simulink model "FCR_sharing"  (R2018a)
settings: Solver=VariableStepAuto  StartTime=0.0  StopTime=25  MaxStep=0.01  RelTol=1e-3
undefined symbols (not defined in the file): Fn, KESS, KGT, Sn, StepMW, Tess, Tgov1, Tgov2
settings Model: Creator=daniemot  LastModifiedBy=daniemot

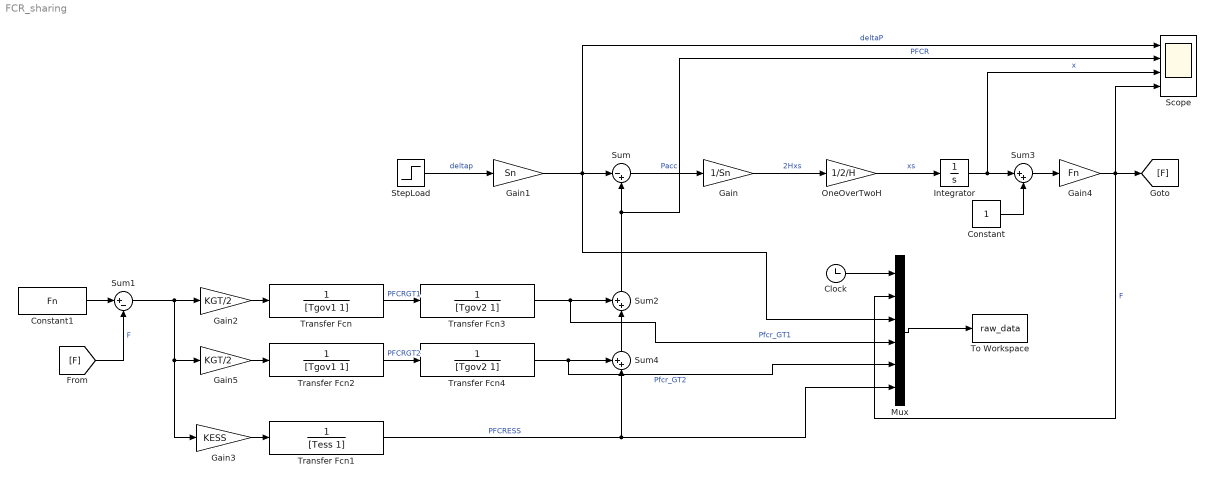
== system FCR_sharing ==
  Clock : Clock
  Constant : Constant
  Constant1 : Constant  Value=Fn
  Gain : Gain  Gain=1/Sn
  Gain1 : Gain  Gain=Sn
  Gain2 : Gain  Gain=KGT/2
  Gain3 : Gain  Gain=KESS
  Gain4 : Gain  Gain=Fn
  Gain5 : Gain  Gain=KGT/2
  Integrator : Integrator
  Mux : Mux  Inputs=6
  OneOverTwoH : Gain  Gain=1/2/H
  Scope : Scope  NumInputPorts=4
  StepLoad : Step  After=StepMW/Sn  SampleTime=0
  Sum : Sum  Inputs=|-+
  Sum1 : Sum  Inputs=|+-
  Sum2 : Sum  Inputs=++|
  Sum3 : Sum  Inputs=|++
  Sum4 : Sum  Inputs=++|
  To Workspace : ToWorkspace  VariableName=raw_data  SampleTime=-1
  Transfer Fcn : TransferFcn  Denominator=[Tgov1 1]
  Transfer Fcn1 : TransferFcn  Denominator=[Tess 1]
  Transfer Fcn2 : TransferFcn  Denominator=[Tgov1 1]
  Transfer Fcn3 : TransferFcn  Denominator=[Tgov2 1]
  Transfer Fcn4 : TransferFcn  Denominator=[Tgov2 1]
  wires:
  OneOverTwoH/1 -> Integrator/1  "xs"
  Gain/1 -> OneOverTwoH/1  "2Hxs"
  Sum/1 -> Gain/1  "Pacc"
  StepLoad/1 -> Gain1/1  "deltap"
  Integrator/1 -> Scope/3, Sum3/1  "x"
  [F] -> Sum1/2  "F"
  Sum1/1 -> Gain2/1, Gain5/1, Gain3/1
  Constant1/1 -> Sum1/1
  Gain2/1 -> Transfer Fcn/1
  Sum2/1 -> Scope/2, Sum/2  "PFCR"
  Gain3/1 -> Transfer Fcn1/1
  Gain4/1 -> Mux/2, Scope/4, [F]  "F"
  Gain1/1 -> Mux/3, Scope/1, Sum/1  "deltaP"
  Sum3/1 -> Gain4/1
  Constant/1 -> Sum3/2
  Sum4/1 -> Sum2/2
  Gain5/1 -> Transfer Fcn2/1
  Transfer Fcn/1 -> Transfer Fcn3/1  "PFCRGT1"
  Transfer Fcn2/1 -> Transfer Fcn4/1  "PFCRGT2"
  Transfer Fcn3/1 -> Mux/4, Sum2/1  "Pfcr_GT1"
  Transfer Fcn4/1 -> Mux/5, Sum4/1  "Pfcr_GT2"
  Transfer Fcn1/1 -> Mux/6, Sum4/2  "PFCRESS"
  Mux/1 -> To Workspace/1
  Clock/1 -> Mux/1
